simulink model "RB_KAIROS_impControl_compensation"  (R2020b)
settings: Solver=ode4  StartTime=0.0  StopTime=t_end  FixedStep=Ts  RelTol=1e-3
values from neighbouring files (symbols this model uses):
  am = 0.3    [RB_KAIROS_ImpControl_OpSpace_quat_2020b_safety_main.m]
  am_r = 0.3    [RB_KAIROS_ImpControl_OpSpace_quat_2020b_safety_main.m]
  Kc = diag(50*ones(6,1))    [RB_KAIROS_ImpControl_OpSpace_quat_2020b_safety_main.m]
  Kp = 2*[400;400;400;400;0;0;0]    [RB_KAIROS_ImpControl_OpSpace_quat_2020b_safety_main.m]
  Kv = [1000;1000;1000;[300;300;300;300;300;300;300]]    [RB_KAIROS_ImpControl_OpSpace_quat_2020b_safety_main.m]
  model_sample_time = 0.001    [RB_KAIROS_ImpControl_OpSpace_quat_2020b_safety_main.m]
  q_dot_0 = zeros(10,1)    [RB_KAIROS_ImpControl_OpSpace_quat_2020b_safety_main.m]
  T_i = K    [RB_KAIROS_ImpControl_OpSpace_quat_2020b_safety_main.m]
  tau_ext = [0 0 0 0 0 0 0 0 0 0 0]    [RB_KAIROS_ImpControl_OpSpace_quat_2020b_safety_main.m]
  v_SMU = 10    [RB_KAIROS_ImpControl_OpSpace_quat_2020b_safety_main.m]
  vm = 0.5    [RB_KAIROS_ImpControl_OpSpace_quat_2020b_safety_main.m]
  vm_r = 0.5    [RB_KAIROS_ImpControl_OpSpace_quat_2020b_safety_main.m]
undefined symbols (not defined in the file or in its folder): DiscIntNeverNeededParam, magnitude, q_0, T_f
libraries: simulink x4, utils x4, transformations_lib x3
(part 16 of 18)

== matlab function RB_KAIROS_impControl_compensation/EE to task space quaternion quantities/MATLAB Function1 ==
  data: R input; qt output
function qt = rotm2quat(R)

qt = rotm2quat(R)';

== matlab function RB_KAIROS_impControl_compensation/EE to task space quaternion quantities/MATLAB Function2 ==
  data: qt input; qt_unit output
function qt_unit = qt_norm(qt)

qt_unit = qt./norm(qt);

== matlab function RB_KAIROS_impControl_compensation/EE to task space quaternion quantities/MATLAB Function4 ==
  data: qt1 input; qt_prod output; qt2 input
function qt_prod = quat_product(qt1,qt2)
% Computes the halmiton product

% Inverse of desired quaternion

eta1 = qt1(1);
eta2 = qt2(1);

eps1 = qt1(2:4);
eps2 = qt2(2:4);

% Quaternion product qt_EE*qt_des_i
qt_prod = [eta1*eta2-dot(eps1,eps2);
    (eta1*eps2+eta2*eps1+cross(eps1,eps2))];

== matlab function RB_KAIROS_impControl_compensation/EE to task space quaternion quantities/Subsystem/S(omega) ==
  data: v input; S output
function S = calc_skewsymm(v)

S = [0 -v(3) v(2);
    v(3) 0 -v(1);
    -v(2) v(1) 0];

== matlab function RB_KAIROS_impControl_compensation/EE to task space quaternion quantities/conjugate ==
  data: qt input; qt_i output
function qt_i = quat_conjugate(qt)

qt_i = [qt(1); -qt(2:4)];
